simulink model "ACS_PIL"  (R2018b)
settings: Solver=FixedStepDiscrete  StartTime=0.0  StopTime=10000  FixedStep=0.01  MaxStep=10  RelTol=1e-5  AbsTol=1e-5  EnableMultiTasking=on
InitFcn:
  | initialization
values from neighbouring files (symbols this model uses):
  A = [0.25  0.25  0.25  0.25  0.25  0.25]    [initialization.m]
  AE = asin(Re/(Re+h))    [initialization.m]
  air_density = [1.2250e+000  3.8990e-002  1.7740e-002  8.2790e-003  3.9720e-003  1.9950e-003  1.0570e-003                5.8210e-004  3.2060e-004  1.7180e-004  8.7700e-005  4.1780e-005  1.9050e-005  8.3370e-006                3.3960e-006  1.3430e-006  5.2970e-007  9.6610e-008  2.4380e-008  8.4840e-009  3.8450e-009                2.0700e-009  1.2440e-009  5.4640e-010  2.7890e-010  7.2480e-011  2.4180e-011  9.1580 ...(+138 chars)    [initialization.m]
  altitude = [    0       25000       30000       35000       40000       45000       50000       55000             60000       65000       70000       75000       80000       85000       90000       95000            100000      110000      120000      130000      140000      150000      160000      180000            200000      250000      300000      350000      400000      450000      500000      600000     ...(+51 chars)    [initialization.m]
  c_diffus = [0.02   0.02   0.02    0.02    0.02    0.02]    [initialization.m]
  c_spec = [0.02   0.02   0.02    0.02    0.02    0.02]    [initialization.m]
  CD = 2    [initialization.m]
  Cell_Area = 30.18*1e-4    (= 0.003018)    [initialization.m]
  CM_mm01 = [-27723, 1088, -239;  -764, -25026, -219; 1299, -416, -23472]    [attitude_control.m]
  CM_mm02 = [-27799, 42,     95; -1261, -26308,  -43; 2693,  458, -24088]    [attitude_control.m]
  CM_mm03 = [9988,0,0; 0, 9989,0; 0,0,10036]    [attitude_control.m]
  CO_mm01 = [2.5332,  2.5200, 2.4915]    [attitude_control.m]
  CO_mm02 = [2.5348,  2.5260, 2.4664]    [attitude_control.m]
  CO_mm03 = [0.0008, -0.0006, 0.0007]    [attitude_control.m]
  cos50 = cos (50/360*2*pi)    [initialization.m]
  cosines = [0.087 0.174  0.500 0.634 0.866]    [initialization.m]
  dip_coel = acos(g01/H0)    [initialization.m]
  dip_long = atan2(h11,g11)    [initialization.m]
  E_EOL = E_BOL*TD_T*TD_R    (= 0.213003)    [initialization.m]
  H0 = norm([g01,g11,h11])    [initialization.m]
  inc = 1.7231    [initialization.m]
  Inertia_tensor = [2.8  0  0;                   0  2.8  0;                   0  0  2]    [initialization.m]
  K_l = 0.1    [initialization.m]
  kelly = [0.000 0.100  0.450 0.635 0.866]    [initialization.m]
  light_speed = 3e8    (= 300000000)    [initialization.m]
  M_SR = 1377*0.967    (= 1331.559)    [initialization.m]
  MM_Working = [1 1 0]    [attitude_control.m]
  N_B = [  1     0    0,         -1     0    0,          0     1    0,          0    -1    0,          0     0    1,          0     0   -1]    [initialization.m]
  Ncell_Xn = 40    [initialization.m]
  Ncell_Xp = 40    [initialization.m]
  Ncell_Yn = 40    [initialization.m]
  Ncell_Yp = 40    [initialization.m]
  Ncell_Zn = 00    (= 0)    [initialization.m]
  Ncell_Zp = 20    [initialization.m]
  NX = [1 0 0]    [initialization.m]
  NY = [0 1 0]    [initialization.m]
  NZ = [0 0 1]    [initialization.m]
  omega_BI_B0 = [0.1;-0.1;-0.1]    [initialization.m]
  omega_e = 7.29e-5    (= 7.29e-05)    [initialization.m]
  omega_o = (1/r)*(G*M/r)^0.5    (= 0.00108253225434)    [initialization.m]
  quat_0 = E321_to_quat([phi0, theta0, psi0])    [initialization.m]
  r = h + Re    (= 6978137)    [initialization.m]
  r_cm_B = [(0.156e-2 * 42.3 + 0.16917 * 22)/64.3,           (0.248e-1 * 42.3 + -0.35948e-1 * 22)/64.3,           (0.164e-2 * 42.3 + 0.14518e-3 * 22)/64.3]    [initialization.m]
  r_cp_a_B = [0 0 0]    [initialization.m]
  r_cp_s_B = [0 0 0]    [initialization.m]
  RAAN_rt = 2.02e-7    (= 2.02e-07)    [initialization.m]
  Re = 6378137    [initialization.m]
  t0 = 2456738.000000    (= 2456738)    [initialization.m]
  TA_0 = 0    [initialization.m]
  theta_g0 = 0    [initialization.m]
undefined symbols (not defined in the file or in its folder): DiscIntNeverNeededParam, magnitude, serial
libraries: simulink x15, vrlib x3, instrumentlib x3, realtime_pacer_lib x1
(part 1 of 3)
settings Model: Creator=assal  LastModifiedBy=jzamora
settings SolverCC: AutoScaleAbsTol=off  ShapePreserveControl=EnableAll  AutoInsertRateTranBlk=on
settings DataIOCC: SaveFormat=Array  SignalLoggingSaveFormat=ModelDataLogs
settings OptimizationCC: BlockReduction=off  DefaultParameterBehavior=Inlined  BufferReuse=off  ExpressionDepthLimit=2147483647  InitFltsAndDblsToZero=on  LifeSpan=inf
settings DebuggingCC: ArtificialAlgebraicLoopMsg=none  CheckSSInitialOutputMsg=off  UnderspecifiedInitializationDetection=Classic  MergeDetectMultiDrivingBlocksExec=none  BlockPriorityViolationMsg=error  SolverPrmCheckMsg=error  Int32ToFloatConvMsg=none  ParameterPrecisionLossMsg=none  ParameterTunabilityLossMsg=none  FcnCallInpInsideContextMsg=warning  StateNameClashWarn=warning  SFUnexpectedBacktrackingDiag=warning  SFNoUnconditionalDefaultTransitionDiag=warning  SFExecutionAtInitializationDiag=none
settings HardwareCC: ProdBitPerPointer=32  ProdBitPerSizeT=32  ProdBitPerPtrDiffT=32  ProdLargestAtomicFloat=None  ProdIntDivRoundTo=Undefined  ProdEndianess=Unspecified  ProdWordSize=32  ProdHWDeviceType=32-bit Generic
settings ModelReferenceCC: PropagateSignalLabelsOutOfModel=off
settings SFSimCC: SimUseLocalCustomCode=off
settings RTWCC: RTWUseLocalCustomCode=off
settings CodeAppCC: StateflowObjectComments=on
settings GRTTargetCC: TargetLangStandard=C89/C90 (ANSI)  GeneratePreprocessorConditionals=Disable all  CombineOutputUpdateFcns=off  GRTInterface=on
settings ConfigComp: CovMetricSettings=dw  CovHtmlReporting=on  CovSaveCumulativeToWorkspaceVar=on  CovSaveSingleToWorkspaceVar=on  CovExternalEMLEnable=off

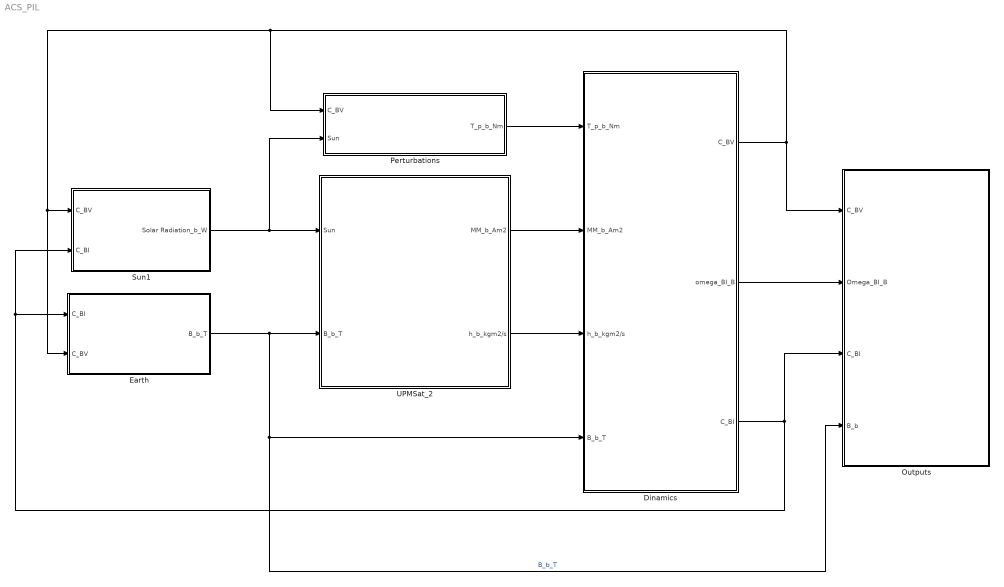
== system ACS_PIL ==
  Dinamics : Subsystem
  Earth : Subsystem
  Outputs : Subsystem
  Perturbations : Subsystem
  Sun1 : Subsystem
  UPMSat_2 : Subsystem
  wires:
  Earth/1(B_b_T) -> Outputs/4(B_b), Dinamics/4(B_b_T), UPMSat_2/2(B_b_T)  "B_b_T"
  Sun1/1(Solar Radiation_b_W) -> Perturbations/2(Sun), UPMSat_2/1(Sun)
  UPMSat_2/1(MM_b_Am2) -> Dinamics/2(MM_b_Am2)
  Perturbations/1(T_p_b_Nm) -> Dinamics/1(T_p_b_Nm)
  Dinamics/1(C_BV) -> Earth/2(C_BV), Sun1/1(C_BV), Perturbations/1(C_BV), Outputs/1(C_BV)
  Dinamics/2(omega_BI_B) -> Outputs/2(Omega_BI_B)
  Dinamics/3(C_BI) -> Outputs/3(C_BI), Earth/1(C_BI), Sun1/2(C_BI)
  UPMSat_2/2(h_b_kgm2/s) -> Dinamics/3(h_b_kgm2/s)

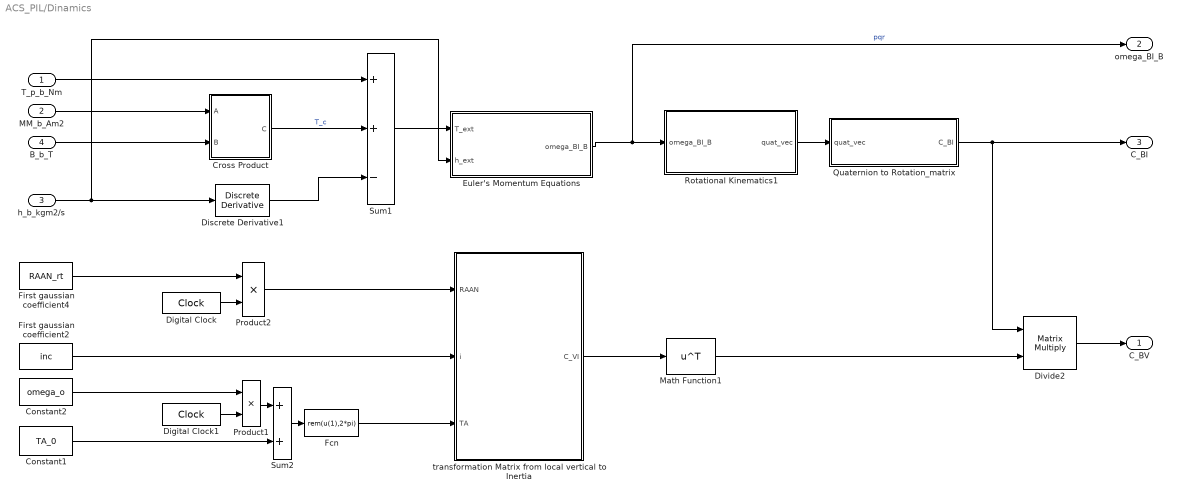
== system ACS_PIL/Dinamics ==
  T_p_b_Nm : Inport
  MM_b_Am2 : Inport  Port=2
  h_b_kgm2/s : Inport  Port=3
  B_b_T : Inport  Port=4
  " First gaussian coefficient2" : Constant  Value=inc
  " First gaussian coefficient4" : Constant  Value=RAAN_rt
  Constant1 : Constant  Value=TA_0
  Constant2 : Constant  Value=omega_o
  Cross Product : Subsystem
  Digital Clock : DigitalClock  SampleTime=0.01
  Digital Clock1 : DigitalClock  SampleTime=0.01
  Discrete Derivative1 : simulink/Discrete/Discrete Derivative  gainval=1.0  ICPrevScaledInput=0.0  OutMin=[]  OutMax=[]  OutDataType=fixdt(1, 16)  OutScaling=2^-10  DoSatur=off
  Divide2 : Product  Inputs=**  Multiplication=Matrix(*)
  Euler's Momentum Equations : Subsystem
  Fcn : Fcn  Expr=rem(u(1),2*pi)
  Math Function1 : Math  Operator=transpose  SaturateOnIntegerOverflow=on
  Product1 : Product  RndMeth=Zero
  Product2 : Product  RndMeth=Zero
  Quaternion to Rotation_matrix : Subsystem
  Rotational Kinematics1 : Subsystem
  Sum1 : Sum  Inputs=++-
  Sum2 : Sum
  transformation Matrix from local vertical to Inertia : Subsystem
  C_BV : Outport
  omega_BI_B : Outport  Port=2
  C_BI : Outport  Port=3
  wires:
  T_p_b_Nm/1 -> Sum1/1
  Sum1/1 -> Euler's Momentum Equations/1(T_ext)
  Euler's Momentum Equations/1(omega_BI_B) -> Rotational Kinematics1/1(omega_BI_B), omega_BI_B/1  "pqr"
  B_b_T/1 -> Cross Product/2(B)
  MM_b_Am2/1 -> Cross Product/1(A)
  Cross Product/1(C) -> Sum1/2  "T_c"
  h_b_kgm2/s/1 -> Discrete Derivative1/1, Euler's Momentum Equations/2(h_ext)
  Rotational Kinematics1/1(quat_vec) -> Quaternion to Rotation_matrix/1(quat_vec)
  Quaternion to Rotation_matrix/1(C_BI) -> Divide2/1, C_BI/1
  Constant2/1 -> Product1/1
  Digital Clock1/1 -> Product1/2
  Product1/1 -> Sum2/1
  Constant1/1 -> Sum2/2
  Sum2/1 -> Fcn/1
  Fcn/1 -> transformation Matrix from local vertical to Inertia/3(TA)
  " First gaussian coefficient4"/1 -> Product2/1
  Digital Clock/1 -> Product2/2
  Product2/1 -> transformation Matrix from local vertical to Inertia/1(RAAN)
  " First gaussian coefficient2"/1 -> transformation Matrix from local vertical to Inertia/2(i)
  transformation Matrix from local vertical to Inertia/1(C_VI) -> Math Function1/1
  Divide2/1 -> C_BV/1
  Math Function1/1 -> Divide2/2
  Discrete Derivative1/1 -> Sum1/3

== system ACS_PIL/Earth ==
  C_BI : Inport
  C_BV : Inport  Port=2
  " First gaussian coefficient1" : Constant  Value=dip_coel
  " First gaussian coefficient3" : Constant  Value=dip_long
  " average rotation rate of the Earth" : Constant  Value=omega_e
  Digital Clock1 : DigitalClock  SampleTime=0.01
  Product5 : Product  RndMeth=Zero
  Simple model of Earth's Magnetic Field1 : Subsystem
  Sum2 : Sum
  greenwich sidereal time : Constant  Value=theta_g0
  transformation Matrix fromEarth Centered to Inertia : Subsystem
  B_b_T : Outport
  wires:
  Digital Clock1/1 -> Product5/1
  transformation Matrix fromEarth Centered to Inertia/1(C_ECEFI) -> Simple model of Earth's Magnetic Field1/5(C_ECEFI)
  greenwich sidereal time/1 -> Sum2/1
  Product5/1 -> Sum2/2
  Sum2/1 -> transformation Matrix fromEarth Centered to Inertia/1(dalpha_g)
  " average rotation rate of the Earth"/1 -> Product5/2
  " First gaussian coefficient3"/1 -> Simple model of Earth's Magnetic Field1/4(phi_md)
  " First gaussian coefficient1"/1 -> Simple model of Earth's Magnetic Field1/3(teta_md)
  Simple model of Earth's Magnetic Field1/1(B_b_T) -> B_b_T/1
  C_BI/1 -> Simple model of Earth's Magnetic Field1/1(C_BI)
  C_BV/1 -> Simple model of Earth's Magnetic Field1/2(C_BV)

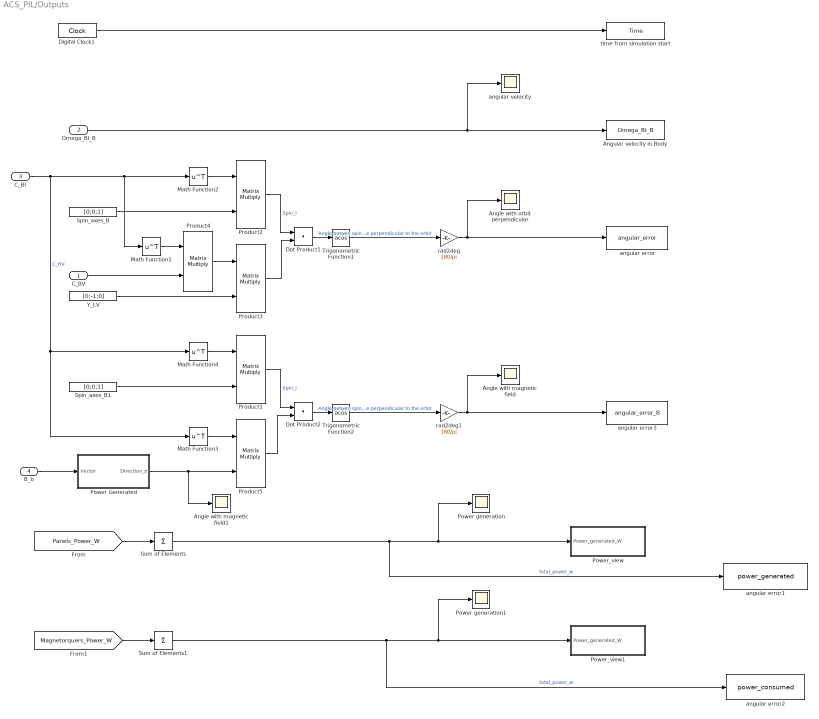
== system ACS_PIL/Outputs ==
  C_BV : Inport
  Omega_BI_B : Inport  Port=2
  C_BI : Inport  Port=3
  B_b : Inport  Port=4
  Angle with magnetic field : Scope
  Angle with magnetic field1 : Scope
  Angle with orbit perpendicular : Scope
  Angular velocity in Body : ToWorkspace  VariableName=Omega_BI_B  SampleTime=-1
      settings: Decimation=1000
  Digital Clock1 : DigitalClock  SampleTime=0.01
  Dot Product1 : DotProduct  InputSameDT=on  OutDataTypeStr=Inherit: Inherit via internal rule
  Dot Product2 : DotProduct  InputSameDT=on  OutDataTypeStr=Inherit: Inherit via internal rule
  Math Function{1..4} (4 alike) : Math  Operator=transpose  SaturateOnIntegerOverflow=on
  Power Generated : Subsystem
  Power generation : Scope
  Power generation1 : Scope
  Power_view : Subsystem
  Power_view1 : Subsystem
  Product{1..5} (5 alike) : Product  Multiplication=Matrix(*)  RndMeth=Zero
  Spin_axes_B : Constant  Value=[0;0;1]
  Spin_axes_B1 : Constant  Value=[0;0;1]
  Sum of Elements : Sum  Inputs=+
  Sum of Elements1 : Sum  Inputs=+
  Trigonometric Function1 : Trigonometry  Operator=acos
  Trigonometric Function2 : Trigonometry  Operator=acos
  Y_LV : Constant  Value=[0;-1;0]
  angular error : ToWorkspace  VariableName=angular_error  SampleTime=-1
      settings: Decimation=1000
  angular error1 : ToWorkspace  VariableName=power_generated  SampleTime=-1
      settings: Decimation=1000
  angular error2 : ToWorkspace  VariableName=power_consumed  SampleTime=-1
      settings: Decimation=1000
  angular error3 : ToWorkspace  VariableName=angular_error_B  SampleTime=-1
      settings: Decimation=1000
  angular velocity : Scope
  rad2deg : Gain  Gain=180/pi
  rad2deg1 : Gain  Gain=180/pi
  time from simulation start : ToWorkspace  VariableName=Time  SampleTime=-1
      settings: Decimation=1000
  wires:
  C_BI/1 -> Math Function3/1, Math Function4/1, Math Function1/1, Math Function2/1  "C_BV"
  Spin_axes_B/1 -> Product2/2
  Product2/1 -> Dot Product1/1  "Spin_I"
  Dot Product1/1 -> Trigonometric Function1/1
  Trigonometric Function1/1 -> rad2deg/1  "Angle betwen spin and the perpendicular to the orbit"
  rad2deg/1 -> angular error/1, Angle with orbit perpendicular/1
  [Panels_Power_W] -> Sum of Elements/1
  Sum of Elements/1 -> angular error1/1, Power generation/1, Power_view/1(Power_generated_W)  "total_power_w"
  Digital Clock1/1 -> time from simulation start/1
  Omega_BI_B/1 -> angular velocity/1, Angular velocity in Body/1
  Math Function2/1 -> Product2/1
  Product3/1 -> Dot Product1/2
  C_BV/1 -> Product4/2
  Math Function1/1 -> Product4/1
  Product4/1 -> Product3/1
  Y_LV/1 -> Product3/2
  [Magnetorquers_Power_W] -> Sum of Elements1/1
  Sum of Elements1/1 -> angular error2/1, Power_view1/1(Power_generated_W), Power generation1/1  "total_power_w"
  Spin_axes_B1/1 -> Product1/2
  Product1/1 -> Dot Product2/1  "Spin_I"
  Dot Product2/1 -> Trigonometric Function2/1
  Trigonometric Function2/1 -> rad2deg1/1  "Angle betwen spin and the perpendicular to the orbit"
  rad2deg1/1 -> Angle with magnetic field/1, angular error3/1
  Math Function4/1 -> Product1/1
  Product5/1 -> Dot Product2/2
  B_b/1 -> Power Generated/1(Vector)
  Math Function3/1 -> Product5/1
  Power Generated/1(Direction_b) -> Angle with magnetic field1/1, Product5/2

== system ACS_PIL/Perturbations ==
  C_BV : Inport
  Sun : Inport  Port=2
  Aerodinamic_Torque : Subsystem
  Gain : Gain
  Gain1 : Gain
  Gain2 : Gain
  Gravity Gradient Torque : Subsystem
  Sum1 : Sum  Inputs=3
  perturbation_Torque1 : Subsystem
  T_p_b_Nm : Outport
  wires:
  Gravity Gradient Torque/1(Tg_B) -> Gain/1
  Aerodinamic_Torque/1(Ta_B) -> Gain1/1
  Gain/1 -> Sum1/1
  Gain1/1 -> Sum1/2
  C_BV/1 -> Aerodinamic_Torque/1(C_BV), Gravity Gradient Torque/1(C_BV)
  Sun/1 -> perturbation_Torque1/1(S_ES_B)
  Sum1/1 -> T_p_b_Nm/1  "T_perturbation_b_Nm"
  perturbation_Torque1/1(Ts_B) -> Gain2/1
  Gain2/1 -> Sum1/3

== system ACS_PIL/Sun1 ==
  C_BV : Inport
  C_BI : Inport  Port=2
  Bus Creator : BusCreator  Inputs=2
  Digital Clock1 : DigitalClock  SampleTime=0.01
  Gain : Gain  Gain=pi/180
  Gain1 : Gain  Gain=pi/180
  Gain2 : Gain  Gain=pi/180
  Min Solar Constant W : Constant  Value=M_SR
  Solar Rays Direction : Subsystem
  Sun Annalema : Subsystem
  Solar Radiation_b_W : Outport
  wires:
  Digital Clock1/1 -> Sun Annalema/1(clock)
  Sun Annalema/2(EOT_deg) -> Gain1/1  "EOT_deg"
  Sun Annalema/3(declination_deg) -> Gain2/1  "declination_deg"
  Gain1/1 -> Solar Rays Direction/3(epsilon)  "EOT_rad"
  Gain2/1 -> Solar Rays Direction/4(delta)  "declination_rad"
  Sun Annalema/1(gamma_deg) -> Gain/1
  Gain/1 -> Solar Rays Direction/2(gamma)
  C_BV/1 -> Solar Rays Direction/5(C_BV)
  Min Solar Constant W/1 -> Solar Rays Direction/1(Solar_const)
  Solar Rays Direction/2(Eclipse) -> Bus Creator/2  "eclipse"
  Solar Rays Direction/1(Sun_b_W) -> Bus Creator/1  "sun_b_W"
  Bus Creator/1 -> Solar Radiation_b_W/1
  C_BI/1 -> Solar Rays Direction/6(C_BI)

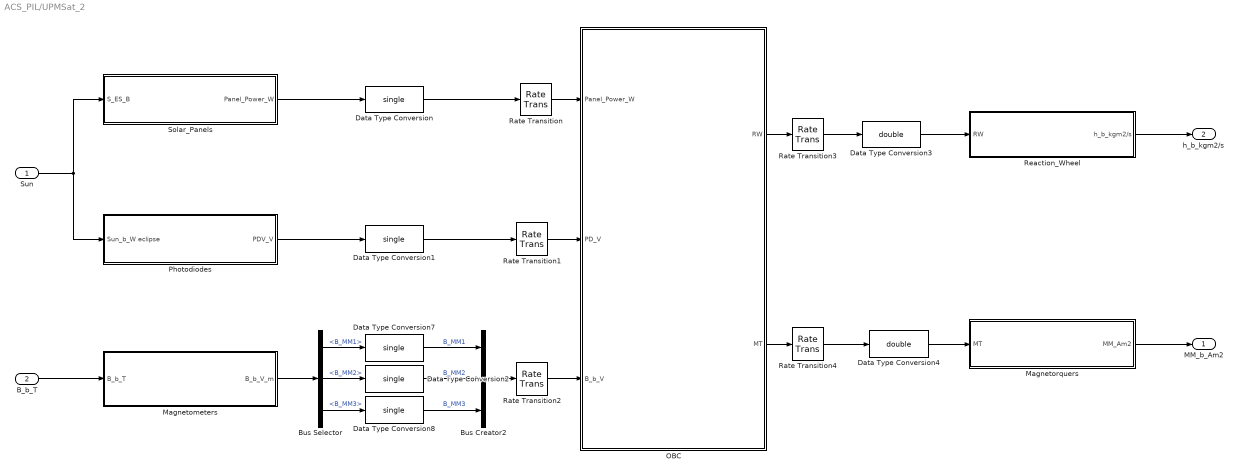
== system ACS_PIL/UPMSat_2 ==
  Sun : Inport
  B_b_T : Inport  Port=2
  Bus Creator2 : BusCreator  Inputs=3
  Bus Selector : BusSelector  OutputSignals=B_MM1,B_MM2,B_MM3
  Data Type Conversion{,1..2,7..8} (5 alike) : DataTypeConversion  OutDataTypeStr=single
  Data Type Conversion3 : DataTypeConversion  OutDataTypeStr=double
  Data Type Conversion4 : DataTypeConversion  OutDataTypeStr=double
  Magnetometers : Subsystem
  Magnetorquers : Subsystem
  OBC : Subsystem
  Photodiodes : Subsystem
  Rate Transition : RateTransition  OutPortSampleTime=0.1
  Rate Transition1 : RateTransition  OutPortSampleTime=0.1
  Rate Transition2 : RateTransition  OutPortSampleTime=0.1
  Rate Transition3 : RateTransition  OutPortSampleTime=0.01
  Rate Transition4 : RateTransition  OutPortSampleTime=0.01
  Reaction_Wheel : Subsystem
  Solar_Panels : Subsystem
  MM_b_Am2 : Outport
  h_b_kgm2/s : Outport  Port=2
  wires:
  Sun/1 -> Solar_Panels/1(S_ES_B), Photodiodes/1(Sun_b_W eclipse)
  Solar_Panels/1(Panel_Power_W) -> Data Type Conversion/1
  Photodiodes/1(PDV_V) -> Data Type Conversion1/1
  Magnetometers/1(B_b_V_m) -> Bus Selector/1
  Reaction_Wheel/1(h_b_kgm2/s) -> h_b_kgm2/s/1
  Magnetorquers/1(MM_Am2) -> MM_b_Am2/1
  B_b_T/1 -> Magnetometers/1(B_b_T)
  Data Type Conversion/1 -> Rate Transition/1
  Data Type Conversion1/1 -> Rate Transition1/1
  Bus Selector/1 -> Data Type Conversion7/1  "<B_MM1>"
  Bus Selector/2 -> Data Type Conversion2/1  "<B_MM2>"
  Bus Selector/3 -> Data Type Conversion8/1  "<B_MM3>"
  Data Type Conversion2/1 -> Bus Creator2/2  "B_MM2"
  Data Type Conversion8/1 -> Bus Creator2/3  "B_MM3"
  Data Type Conversion7/1 -> Bus Creator2/1  "B_MM1"
  Bus Creator2/1 -> Rate Transition2/1
  Data Type Conversion3/1 -> Reaction_Wheel/1(RW)
  Data Type Conversion4/1 -> Magnetorquers/1(MT)
  OBC/2(MT) -> Rate Transition4/1
  OBC/1(RW) -> Rate Transition3/1
  Rate Transition/1 -> OBC/1(Panel_Power_W)
  Rate Transition1/1 -> OBC/2(PD_V)
  Rate Transition2/1 -> OBC/3(B_b_V)
  Rate Transition3/1 -> Data Type Conversion3/1
  Rate Transition4/1 -> Data Type Conversion4/1

== system ACS_PIL/Dinamics/Cross Product ==
  A : Inport
  B : Inport  Port=2
  Cross Product : Fcn  Expr=u(2)*u(6)-u(3)*u(5)
  Cross Product1 : Fcn  Expr=u(3)*u(4)-u(1)*u(6)
  Cross Product2 : Fcn  Expr=u(1)*u(5)-u(2)*u(4)
  Mux : Mux  Inputs=2
  Mux1 : Mux  Inputs=3
  C : Outport
  wires:
  A/1 -> Mux/1
  B/1 -> Mux/2
  Mux1/1 -> C/1
  Mux/1 -> Cross Product2/1, Cross Product1/1, Cross Product/1
  Cross Product1/1 -> Mux1/2
  Cross Product2/1 -> Mux1/3
  Cross Product/1 -> Mux1/1

== system ACS_PIL/Dinamics/Euler's Momentum Equations ==
  T_ext : Inport
  h_ext : Inport  Port=2
  Add1 : Sum  Inputs=-+
  Add2 : Sum  Inputs=2
  Constant : Constant  Value=Inertia_tensor  VectorParams1D=off
  Constant1 : Constant  Value=omega_BI_B0  VectorParams1D=off
  Cross Product : Subsystem
  Discrete-Time Integrator : DiscreteIntegrator  InitialConditionSource=external  SampleTime=0.01  ICPrevOutput=DiscIntNeverNeededParam  ICPrevScaledInput=DiscIntNeverNeededParam
  Product : Product  Inputs=/  Multiplication=Matrix(*)
  Product1 : Product  Multiplication=Matrix(*)  RndMeth=Zero
  Product2 : Product  Multiplication=Matrix(*)  RndMeth=Zero
  omega_BI_B : Outport
  wires:
  Product1/1 -> Add2/1  "I * omega_BI_B"
  Product2/1 -> Discrete-Time Integrator/1  "omega_BI_B_dot"
  Add1/1 -> Product2/2
  Product/1 -> Product2/1
  T_ext/1 -> Add1/2
  Cross Product/1(C) -> Add1/1
  Discrete-Time Integrator/1 -> Cross Product/1(A), Product1/2, omega_BI_B/1  "omega_BI_B"
  Constant/1 -> Product/1, Product1/1
  Add2/1 -> Cross Product/2(B)
  h_ext/1 -> Add2/2
  Constant1/1 -> Discrete-Time Integrator/2

== system ACS_PIL/Dinamics/Quaternion to Rotation_matrix ==
  quat_vec : Inport
  Fcn : Fcn  Expr=1-2*(u(2)^2+u(3)^2)
  Fcn1 : Fcn  Expr=2*(u(1)*u(2)-u(3)*u(4))
  Fcn2 : Fcn  Expr=2*(u(1)*u(3)+u(2)*u(4))
  Fcn3 : Fcn  Expr=2*(u(1)*u(2)+u(3)*u(4))
  Fcn4 : Fcn  Expr=1-2*(u(1)^2+u(3)^2)
  Fcn5 : Fcn  Expr=2*(u(2)*u(3)-u(4)*u(1))
  Fcn6 : Fcn  Expr=2*(u(1)*u(3)-u(4)*u(2))
  Fcn7 : Fcn  Expr=2*(u(2)*u(3)+u(4)*u(1))
  Fcn8 : Fcn  Expr=1-2*(u(1)^2+u(2)^2)
  Mux : Mux  Inputs=9
  Reshape : Reshape  OutputDimensionality=Customize  OutputDimensions=[3,3]
  C_BI : Outport
  wires:
  Reshape/1 -> C_BI/1
  Mux/1 -> Reshape/1
  Fcn8/1 -> Mux/9
  Fcn7/1 -> Mux/8
  Fcn6/1 -> Mux/7
  Fcn5/1 -> Mux/6
  Fcn4/1 -> Mux/5
  Fcn3/1 -> Mux/4
  Fcn2/1 -> Mux/3
  Fcn1/1 -> Mux/2
  Fcn/1 -> Mux/1
  quat_vec/1 -> Fcn8/1, Fcn7/1, Fcn6/1, Fcn5/1, Fcn4/1, Fcn3/1, Fcn2/1, Fcn1/1, Fcn/1

== system ACS_PIL/Dinamics/Rotational Kinematics1 ==
  omega_BI_B : Inport
  4*4 Skew Mtrix of a 3*1 vector : Subsystem
  Constant : Constant  Value=quat_0
  Constant1 : Constant
  Constant2 : Constant  Value=K_l
  Discrete-Time Integrator : DiscreteIntegrator  InitialConditionSource=external  SampleTime=0.01  ICPrevOutput=DiscIntNeverNeededParam  ICPrevScaledInput=DiscIntNeverNeededParam
  Divide1 : Product  Inputs=*/
  Divide3 : Product  Inputs=3
  Gain : Gain  Gain=1/2
  Math Function : Math  Operator=magnitude^2  SaturateOnIntegerOverflow=on
  Product : Product  Multiplication=Matrix(*)  RndMeth=Zero
  Quaternion Norm : Subsystem  AncestorBlock=aerolibutil/Quaternion Norm  mask(Quaternion Norm){}
      mask help: Calculate the norm of a quaternion.
      mask Help: web(asbhelp);
  Quaternion Norm1 : Subsystem  AncestorBlock=aerolibutil/Quaternion Norm  mask(Quaternion Norm){}
      mask help: Calculate the norm of a quaternion.
      mask Help: web(asbhelp);
  Sum : Sum  Inputs=+-
  Sum2 : Sum
  quat_vec : Outport
  wires:
  Quaternion Norm1/1(norm(q)) -> Math Function/1
  Divide1/1 -> Quaternion Norm1/1(q), Divide3/2, Product/2, quat_vec/1
  Divide3/1 -> Sum2/2
  Gain/1 -> Sum2/1
  Constant2/1 -> Divide3/1
  Sum2/1 -> Discrete-Time Integrator/1
  Constant/1 -> Discrete-Time Integrator/2
  Sum/1 -> Divide3/3  "epsilon_t"
  Math Function/1 -> Sum/2
  Constant1/1 -> Sum/1
  Product/1 -> Gain/1
  Quaternion Norm/1(norm(q)) -> Divide1/2
  omega_BI_B/1 -> 4*4 Skew Mtrix of a 3*1 vector/1(omega)
  Discrete-Time Integrator/1 -> Divide1/1, Quaternion Norm/1(q)
  4*4 Skew Mtrix of a 3*1 vector/1(4*4 omega_skew matrix1) -> Product/1

== system ACS_PIL/Dinamics/transformation Matrix from local vertical to Inertia ==
  RAAN : Inport
  i : Inport  Port=2
  TA : Inport  Port=3
  Inertial 2 Orbital Plane1 : Subsystem
  Orbital Reference 2 Local Vertical1 : Subsystem
  Product : Product  Multiplication=Matrix(*)  RndMeth=Zero
  Product1 : Product  Multiplication=Matrix(*)  RndMeth=Zero
  C_VI : Outport
  wires:
  Inertial 2 Orbital Plane1/1(C_OPROPF) -> Product/2  "C_OPROPF"
  Orbital Reference 2 Local Vertical1/1(C_VOPR) -> Product/1  "C_VOPR"
  TA/1 -> Inertial 2 Orbital Plane1/3(TA)
  RAAN/1 -> Inertial 2 Orbital Plane1/2(RAAN)
  i/1 -> Inertial 2 Orbital Plane1/1(i)
  Product/1 -> Product1/1
  Product1/1 -> C_VI/1
  Inertial 2 Orbital Plane1/2(C_OPFI) -> Product1/2  "C_OPFI"

== system ACS_PIL/Earth/Simple model of Earth's Magnetic Field1 ==
  C_BI : Inport
  C_BV : Inport  Port=2
  teta_md : Inport  Port=3
  phi_md : Inport  Port=4
  C_ECEFI : Inport  Port=5
  Demux : Demux  Outputs=2
  Divide1 : Product  Inputs=**  Multiplication=Matrix(*)
  Divide10 : Product  Inputs=**  Multiplication=Matrix(*)
  Math Function1 : Math  Operator=transpose  SaturateOnIntegerOverflow=on
  Math Function2 : Math  Operator=transpose  SaturateOnIntegerOverflow=on
  Product1 : Product  Multiplication=Matrix(*)  RndMeth=Zero
  Product4 : Product  Inputs=3  Multiplication=Matrix(*)  RndMeth=Zero
  Simple model of Earth's Magnetic Field1 : Subsystem
  earth_sat vector in local vertical reference system : Constant  Value=[0 ;0 ;-r]  VectorParams1D=off
  longitude_latitude : Subsystem
  B_b_T : Outport
  wires:
  teta_md/1 -> Simple model of Earth's Magnetic Field1/3(teta_md)
  phi_md/1 -> Simple model of Earth's Magnetic Field1/4(phi_md)
  longitude_latitude/1(long_lat) -> Demux/1
  Demux/1 -> Simple model of Earth's Magnetic Field1/1(long)
  Demux/2 -> Simple model of Earth's Magnetic Field1/2(lat)
  earth_sat vector in local vertical reference system/1 -> Divide10/2  "R_LV"
  Divide10/1 -> longitude_latitude/1(R_ECEF)  "R_ECEF"
  Product4/1 -> Divide10/1  "C_ECEFV"
  C_BV/1 -> Product4/3
  Math Function2/1 -> Product4/2
  C_BI/1 -> Math Function2/1, Product1/1
  Divide1/1 -> B_b_T/1
  C_ECEFI/1 -> Math Function1/1, Product4/1
  Product1/1 -> Divide1/1  "C_BECEF"
  Simple model of Earth's Magnetic Field1/1(B_ECEF_T) -> Divide1/2
  Math Function1/1 -> Product1/2

== system ACS_PIL/Earth/transformation Matrix fromEarth Centered to Inertia ==
  dalpha_g : Inport
  Constant{1,4..5,8} (4 alike) : Constant  Value=0
  Constant6 : Constant
  Gain : Gain  Gain=-1
  Mux : Mux  Inputs=9
  Reshape : Reshape  OutputDimensionality=Customize  OutputDimensions=[3,3]
  Trigonometric Function : Trigonometry  Operator=cos
  Trigonometric Function1 : Trigonometry
  C_ECEFI : Outport
  wires:
  Mux/1 -> Reshape/1
  Trigonometric Function1/1 -> Gain/1, Mux/4
  Constant1/1 -> Mux/3
  Constant5/1 -> Mux/6
  Constant8/1 -> Mux/7
  Constant4/1 -> Mux/8
  Constant6/1 -> Mux/9
  Reshape/1 -> C_ECEFI/1
  Trigonometric Function/1 -> Mux/1, Mux/5
  dalpha_g/1 -> Trigonometric Function1/1, Trigonometric Function/1
  Gain/1 -> Mux/2

== system ACS_PIL/Outputs/Power Generated ==
  Vector : Inport
  Add : Sum  Inputs=+++
  Add1 : Sum  Inputs=2
  Compare To Zero : simulink/Logic and Bit Operations/Compare To Zero  relop===  OutDataTypeStr=uint8  ZeroCross=off
  Demux : Demux  Outputs=3
  Math Function : Math  Operator=magnitude^2  SaturateOnIntegerOverflow=on
  Math Function1 : Math  Operator=magnitude^2  SaturateOnIntegerOverflow=on
  Math Function2 : Math  Operator=magnitude^2  SaturateOnIntegerOverflow=on
  Math Function3 : Math  Operator=sqrt  SaturateOnIntegerOverflow=on
  Product4 : Product  Inputs=*/  RndMeth=Zero
  Direction_b : Outport
  wires:
  Demux/1 -> Math Function/1
  Demux/2 -> Math Function1/1
  Math Function/1 -> Add/1
  Math Function1/1 -> Add/2
  Add/1 -> Math Function3/1
  Math Function3/1 -> Add1/1, Compare To Zero/1
  Demux/3 -> Math Function2/1
  Math Function2/1 -> Add/3
  Vector/1 -> Product4/1, Demux/1
  Product4/1 -> Direction_b/1
  Add1/1 -> Product4/2
  Compare To Zero/1 -> Add1/2

== system ACS_PIL/Outputs/Power_view ==
  Power_generated_W : Inport
  Discrete-Time Integrator : DiscreteIntegrator  SampleTime=0.01  ICPrevOutput=DiscIntNeverNeededParam  ICPrevScaledInput=DiscIntNeverNeededParam
  Product : Product  Inputs=*/  RndMeth=Zero
  Ramp : simulink/Sources/Ramp  slope=1  start=0  InitialOutput=0.001
  Terminator1 : Terminator
  wires:
  Discrete-Time Integrator/1 -> Product/1
  Ramp/1 -> Product/2
  Power_generated_W/1 -> Discrete-Time Integrator/1
  Product/1 -> Terminator1/1

== system ACS_PIL/Outputs/Power_view1 ==
  Power_generated_W : Inport
  Discrete-Time Integrator : DiscreteIntegrator  SampleTime=0.01  ICPrevOutput=DiscIntNeverNeededParam  ICPrevScaledInput=DiscIntNeverNeededParam
  Product : Product  Inputs=*/  RndMeth=Zero
  Ramp : simulink/Sources/Ramp  slope=1  start=0  InitialOutput=0.001
  Terminator1 : Terminator
  wires:
  Product/1 -> Terminator1/1
  Power_generated_W/1 -> Discrete-Time Integrator/1
  Ramp/1 -> Product/2
  Discrete-Time Integrator/1 -> Product/1

== system ACS_PIL/Perturbations/Aerodinamic_Torque ==
  C_BV : Inport
  Add3 : Sum  Inputs=+-
  Aerodynamic : Subsystem
  Earth's radius : Constant  Value=Re
  Subsystem : Subsystem
  air_density1 : Lookup  InputValues=altitude  Table=air_density
  r_sat : Constant  Value=r
  Ta_B : Outport
  wires:
  Subsystem/1(v_vec_b) -> Aerodynamic/1(v_B)
  r_sat/1 -> Add3/1
  Earth's radius/1 -> Add3/2
  Add3/1 -> air_density1/1
  air_density1/1 -> Aerodynamic/2(air_density)
  C_BV/1 -> Subsystem/1(C_BV)
  Aerodynamic/1(Ta_B) -> Ta_B/1

== system ACS_PIL/Perturbations/Gravity Gradient Torque ==
  C_BV : Inport
  Constant1 : Constant  Value=Inertia_tensor
  Constant2 : Constant  Value=omega_o
  Constant4 : Constant  Value=3  VectorParams1D=off
  Cross Product : vrlib/Utilities/Cross Product
      settings: SourceProductBaseCode=VR
  Divide : Product  Inputs=***
  Math Function : Math  Operator=square  SaturateOnIntegerOverflow=on
  Product : Product  Multiplication=Matrix(*)  RndMeth=Zero
  Product1 : Product  Multiplication=Matrix(*)  RndMeth=Zero
  sat_earth vector in local vertical reference system : Constant  Value=[0 ;0 ;1]  VectorParams1D=off
  Tg_B : Outport
  wires:
  Math Function/1 -> Divide/3
  Constant2/1 -> Math Function/1
  Divide/1 -> Tg_B/1
  Cross Product/1 -> Divide/1
  Product/1 -> Cross Product/2
  sat_earth vector in local vertical reference system/1 -> Product1/2
  C_BV/1 -> Product1/1
  Product1/1 -> Cross Product/1, Product/2
  Constant1/1 -> Product/1
  Constant4/1 -> Divide/2

== system ACS_PIL/Perturbations/perturbation_Torque1 ==
  S_ES_B : Inport
  Bus Selector : BusSelector  OutputSignals=sun_b_W,eclipse
  Power Generated : Subsystem
  Solar Torque and Force Calculation : Subsystem
  Ts_B : Outport
  wires:
  Bus Selector/2 -> Solar Torque and Force Calculation/3(eclipse)  "<eclipse>"
  Power Generated/2(Solar_Flux_W) -> Solar Torque and Force Calculation/2(Solar_const)
  Power Generated/1(Solar_Direction_b) -> Solar Torque and Force Calculation/1(S_ES_B)
  S_ES_B/1 -> Bus Selector/1
  Bus Selector/1 -> Power Generated/1(Sol_b_W)  "<sun_b_W>"
  Solar Torque and Force Calculation/1(Ts_B) -> Ts_B/1

== system ACS_PIL/Sun1/Solar Rays Direction ==
  Solar_const : Inport
  gamma : Inport  Port=2
  epsilon : Inport  Port=3
  delta : Inport  Port=4
  C_BV : Inport  Port=5
  C_BI : Inport  Port=6
  Divide1 : Product  Inputs=**  Multiplication=Matrix(*)
  Eclipse_ : Subsystem
  Logical Operator : Logic  Operator=NOT  AllPortsSameDT=off  OutDataTypeStr=boolean
  Product8 : Product  RndMeth=Zero
  Solar direction in inertial : Subsystem
  Sun_b_W : Outport
  Eclipse : Outport  Port=2
  wires:
  C_BV/1 -> Eclipse_/2(C_BV)
  Solar direction in inertial/1(S_ES_I) -> Divide1/2
  gamma/1 -> Solar direction in inertial/3(gamma)
  epsilon/1 -> Solar direction in inertial/2(epsilon)
  delta/1 -> Solar direction in inertial/1(delta)
  Solar_const/1 -> Product8/1
  Eclipse_/1(eclipse) -> Logical Operator/1
  Logical Operator/1 -> Eclipse/1
  Divide1/1 -> Eclipse_/1(Earth-Sun B), Product8/2  "Solar radiation direction in body"
  Product8/1 -> Sun_b_W/1
  C_BI/1 -> Divide1/1

== system ACS_PIL/Sun1/Sun Annalema ==
  clock : Inport
  Calculating Sun position : Subsystem  mask(Calculating sun position){}
      mask help:
      | This block calculates the coordinates of the Sun following the specifications in "The astronomical Almanac for the year 2008" in section C24
      | This formulas have a precision of 0.1 minutes from 1950 to 2050.
      |
      | Mean longitude (gamma angle) which is the angle between Vernal equinox and Mean Sun
      | vector. This angle is zero at vernal equiniox (22th of March) and reaches 360deg after a year.
      |
      | Declination (delta) is the angle of the sun respect to the ecuatorial plane of the Earth.
      |
      | Equation of time is the apparent time of the sun minus the mean time (*4 in degrees).
  J2000.0 : Constant  Value=2451545.0
  Sum1 : Sum  Inputs=+-
  Sum2 : Sum
  sec to day : Gain  Gain=1/(24*3600)
  t0 : Constant  Value=t0
  gamma_deg : Outport
  EOT_deg : Outport  Port=2
  declination_deg : Outport  Port=3
  wires:
  J2000.0/1 -> Sum1/2
  clock/1 -> sec to day/1
  sec to day/1 -> Sum2/1
  Sum2/1 -> Sum1/1
  t0/1 -> Sum2/2
  Sum1/1 -> Calculating Sun position/1(Time_passed from J2000.0)  "n of days from J2000.0"
  Calculating Sun position/1(gamma_deg) -> gamma_deg/1
  Calculating Sun position/2(EOT_deg) -> EOT_deg/1
  Calculating Sun position/3(declination_deg) -> declination_deg/1

== system ACS_PIL/UPMSat_2/Magnetometers ==
  B_b_T : Inport
  Bus Creator : BusCreator  Inputs=3
  Gain1 : Gain  Gain=1e9
  Magnetometer_1 : Subsystem
  Magnetometer_2 : Subsystem
  Magnetometer_3 : Subsystem
  B_b_V_m : Outport
  wires:
  B_b_T/1 -> Gain1/1
  Magnetometer_1/1(B_b_V_m1) -> Bus Creator/1  "B_MM1"
  Magnetometer_2/1(B_b_V_m1) -> Bus Creator/2  "B_MM2"
  Magnetometer_3/1(B_b_V_m1) -> Bus Creator/3  "B_MM3"
  Bus Creator/1 -> B_b_V_m/1
  Gain1/1 -> Magnetometer_1/1(B_b_nT), Magnetometer_3/1(B_b_nT), Magnetometer_2/1(B_b_nT)  "B_b_nT"

== system ACS_PIL/UPMSat_2/Magnetorquers ==
  MT : Inport
  Demux2 : Demux  Outputs=3
  Gain1 : Gain  Gain=22
  Gain2 : Gain  Gain=22
  Gain3 : Gain  Gain=22
  Magnetorquers1 : Subsystem
  Magnetorquers2 : Subsystem
  Magnetorquers4 : Subsystem
  Mux : Mux  Inputs=3
  Mux1 : Mux  Inputs=3
  Scope : Scope
  MM_Am2 : Outport
  tag scope: Magnetorquers_Power_W=global
  wires:
  Demux2/1 -> Gain3/1
  Demux2/2 -> Gain1/1
  Demux2/3 -> Gain2/1
  Magnetorquers4/1(MM_Am2) -> Scope/1, Mux/1
  Magnetorquers1/1(MM_Am2) -> Mux/2
  Magnetorquers2/1(MM_Am2) -> Mux/3
  Mux/1 -> MM_Am2/1
  MT/1 -> Demux2/1  "total_power_w"
  Magnetorquers4/2(MM_W) -> Mux1/1
  Magnetorquers1/2(MM_W) -> Mux1/2
  Magnetorquers2/2(MM_W) -> Mux1/3
  Mux1/1 -> [Magnetorquers_Power_W]
  Gain3/1 -> Magnetorquers4/1(MT)
  Gain1/1 -> Magnetorquers1/1(MT)
  Gain2/1 -> Magnetorquers2/1(MT)

== system ACS_PIL/UPMSat_2/OBC ==
  Panel_Power_W : Inport
  PD_V : Inport  Port=2
  B_b_V : Inport  Port=3
  Bus Creator : BusCreator  Inputs=2
  Bus Creator1 : BusCreator  Inputs=2
  Bus Selector : BusSelector  OutputSignals=signal1,signal2
  Bus Selector1 : BusSelector  OutputSignals=signal1,signal2,signal3
  Constant3 : Constant  Value=0  OutDataTypeStr=single
  Data Adquisition : Subsystem
  Experimentall Attitude Control : Subsystem
  Nominal Attitude Control : Subsystem
  Terminator1 : Terminator
  RW : Outport
  MT : Outport  Port=2
  wires:
  B_b_V/1 -> Data Adquisition/3(B_b_V)
  Panel_Power_W/1 -> Data Adquisition/1(PP_W)
  PD_V/1 -> Data Adquisition/2(PD_V)
  Data Adquisition/1(PP_UPC) -> Experimentall Attitude Control/1(PP_UPC)
  Data Adquisition/2(PD_UPC) -> Experimentall Attitude Control/2(PD_UPC)
  Nominal Attitude Control/1(MT) -> Bus Creator/1
  Bus Creator1/1 -> Terminator1/1
  Experimentall Attitude Control/1(MT) -> Bus Creator1/1
  Experimentall Attitude Control/2(RW) -> Bus Creator1/2
  Bus Creator/1 -> Bus Selector/1
  Bus Selector/1 -> MT/1  "<signal1>"
  Bus Selector/2 -> RW/1  "<signal2>"
  Constant3/1 -> Bus Creator/2
  Bus Selector1/2 -> Nominal Attitude Control/2(B_b_mm02_UPC)  "<signal2>"
  Bus Selector1/1 -> Nominal Attitude Control/1(B_b_mm01_UPC)  "<signal1>"
  Bus Selector1/3 -> Nominal Attitude Control/3(B_b_mm03_UPC)  "<signal3>"
  Data Adquisition/3(B_b_UPC) -> Experimentall Attitude Control/3(B_b_UPC), Bus Selector1/1

== system ACS_PIL/UPMSat_2/Photodiodes ==
  Sun_b_W eclipse : Inport
  1 Hz2 : DiscretePulseGenerator  PulseType=Time based  PulseWidth=50
  1 Hz3 : DiscretePulseGenerator  PulseType=Time based  Period=0.2  PulseWidth=50  PhaseDelay=1
  Bus Selector : BusSelector  OutputSignals=sun_b_W,eclipse
  Measurements : Subsystem
  Product1 : Product  RndMeth=Zero
  Sun : Subsystem
  Voltage : Subsystem
  PDV_V : Outport
  wires:
  Voltage/1(PD_V) -> Measurements/1(V)
  Sun_b_W eclipse/1 -> Bus Selector/1
  Bus Selector/1 -> Sun/1(Sol_b_W)  "<sun_b_W>"
  Sun/1(Solar_Direction_b) -> Voltage/1(Earth-Sun B)
  Sun/2(Solar_Flux_W) -> Voltage/2(Solar Constant)
  Bus Selector/2 -> Voltage/3(eclipse)  "<eclipse>"
  Product1/1 -> Measurements/Trigger
  Measurements/1(V_V) -> PDV_V/1
  1 Hz3/1 -> Product1/2
  1 Hz2/1 -> Product1/1

== system ACS_PIL/UPMSat_2/Reaction_Wheel ==
  RW : Inport
  Magnetorquer Fil1 : Constant  Value=0  SampleTime=0.01
  Terminator : Terminator
  h_b_kgm2/s : Outport
  wires:
  RW/1 -> Terminator/1
  Magnetorquer Fil1/1 -> h_b_kgm2/s/1

== system ACS_PIL/UPMSat_2/Solar_Panels ==
  S_ES_B : Inport
  3.33 Hz : DiscretePulseGenerator  PulseType=Time based  Period=0.3  PulseWidth=100-1/0.3
  Bus Selector : BusSelector  OutputSignals=sun_b_W,eclipse
  Measurements : Subsystem
  Power : Subsystem
  Power Generated : Subsystem
  Panel_Power_W : Outport
  tag scope: Panels_Power_W=global
  wires:
  Power/1(Power_each_W) -> [Panels_Power_W], Measurements/1(V)
  Bus Selector/1 -> Power Generated/1(Sol_b_W)  "<sun_b_W>"
  Power Generated/1(Solar_Direction_b) -> Power/1(Earth-Sun B)
  Power Generated/2(Solar_Flux_W) -> Power/2(Solar Constant)
  S_ES_B/1 -> Bus Selector/1
  Bus Selector/2 -> Power/3(eclipse)  "<eclipse>"
  3.33 Hz/1 -> Measurements/Trigger
  Measurements/1(V_V) -> Panel_Power_W/1

== system ACS_PIL/Dinamics/Euler's Momentum Equations/Cross Product ==
  A : Inport
  B : Inport  Port=2
  Cross Product : Fcn  Expr=u(2)*u(6)-u(3)*u(5)
  Cross Product1 : Fcn  Expr=u(3)*u(4)-u(1)*u(6)
  Cross Product2 : Fcn  Expr=u(1)*u(5)-u(2)*u(4)
  Mux : Mux  Inputs=2
  Mux1 : Mux  Inputs=3
  C : Outport
  wires:
  A/1 -> Mux/1
  B/1 -> Mux/2
  Mux1/1 -> C/1
  Mux/1 -> Cross Product2/1, Cross Product1/1, Cross Product/1
  Cross Product1/1 -> Mux1/2
  Cross Product2/1 -> Mux1/3
  Cross Product/1 -> Mux1/1

== system ACS_PIL/Dinamics/Rotational Kinematics1/4*4 Skew Mtrix of a 3*1 vector ==
  omega : Inport
  Constant{,1..3} (4 alike) : Constant  Value=0
  Demux : Demux  Outputs=3
  Demux1 : Demux  Outputs=3
  Gain : Gain  Gain=-1
  Mux1 : Mux  Inputs=16
  Reshape : Reshape  OutputDimensionality=Customize  OutputDimensions=[4,4]
  4*4 omega_skew matrix1 : Outport
  wires:
  omega/1 -> Demux/1, Gain/1
  Gain/1 -> Demux1/1
  Constant/1 -> Mux1/1
  Demux1/3 -> Mux1/2, Mux1/12  "-omega_z"
  Demux/2 -> Mux1/3, Mux1/14  "omega_y"
  Demux/3 -> Mux1/15, Mux1/5  "omega_z"
  Constant1/1 -> Mux1/6
  Demux1/1 -> Mux1/4, Mux1/7  "-omega_x"
  Demux1/2 -> Mux1/8, Mux1/9  "-omega_y"
  Demux/1 -> Mux1/10, Mux1/13  "omega_x"
  Constant2/1 -> Mux1/11
  Constant3/1 -> Mux1/16
  Mux1/1 -> Reshape/1
  Reshape/1 -> 4*4 omega_skew matrix1/1

== system ACS_PIL/Dinamics/Rotational Kinematics1/Quaternion Norm ==
  q : Inport
  Demux : Demux
  Math Function : Math  Operator=sqrt  SaturateOnIntegerOverflow=on
  Product{,1..3} (4 alike) : Product
  Sum : Sum  Inputs=4
  norm(q) : Outport
  wires:
  Demux/4 -> Product3/1, Product3/2
  Demux/3 -> Product2/1, Product2/2
  Demux/2 -> Product1/1, Product1/2
  Demux/1 -> Product/1, Product/2
  Product3/1 -> Sum/4
  Product2/1 -> Sum/3
  Product1/1 -> Sum/2
  Product/1 -> Sum/1
  Sum/1 -> Math Function/1
  q/1 -> Demux/1
  Math Function/1 -> norm(q)/1

== system ACS_PIL/Dinamics/Rotational Kinematics1/Quaternion Norm1 ==
  q : Inport
  Demux : Demux
  Math Function : Math  Operator=sqrt  SaturateOnIntegerOverflow=on
  Product{,1..3} (4 alike) : Product
  Sum : Sum  Inputs=4
  norm(q) : Outport
  wires:
  Math Function/1 -> norm(q)/1
  q/1 -> Demux/1
  Sum/1 -> Math Function/1
  Product/1 -> Sum/1
  Product1/1 -> Sum/2
  Product2/1 -> Sum/3
  Product3/1 -> Sum/4
  Demux/1 -> Product/2, Product/1
  Demux/2 -> Product1/2, Product1/1
  Demux/3 -> Product2/2, Product2/1
  Demux/4 -> Product3/2, Product3/1

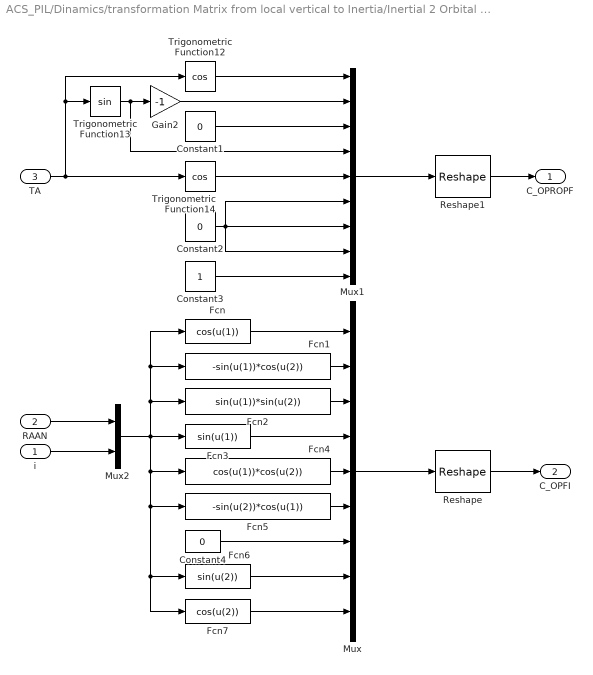
== system ACS_PIL/Dinamics/transformation Matrix from local vertical to Inertia/Inertial 2 Orbital Plane1 ==
  i : Inport
  RAAN : Inport  Port=2
  TA : Inport  Port=3
  Constant1 : Constant  Value=0
  Constant2 : Constant  Value=0
  Constant3 : Constant
  Constant4 : Constant  Value=0
  Fcn : Fcn  Expr=cos(u(1))
  Fcn1 : Fcn  Expr=-sin(u(1))*cos(u(2))
  Fcn2 : Fcn  Expr=sin(u(1))*sin(u(2))
  Fcn3 : Fcn  Expr=sin(u(1))
  Fcn4 : Fcn  Expr=cos(u(1))*cos(u(2))
  Fcn5 : Fcn  Expr=-sin(u(2))*cos(u(1))
  Fcn6 : Fcn  Expr=sin(u(2))
  Fcn7 : Fcn  Expr=cos(u(2))
  Gain2 : Gain  Gain=-1
  Mux : Mux  Inputs=9
  Mux1 : Mux  Inputs=9
  Mux2 : Mux  Inputs=2
  Reshape : Reshape  OutputDimensionality=Customize  OutputDimensions=[3,3]
  Reshape1 : Reshape  OutputDimensionality=Customize  OutputDimensions=[3,3]
  Trigonometric Function12 : Trigonometry  Operator=cos
  Trigonometric Function13 : Trigonometry
  Trigonometric Function14 : Trigonometry  Operator=cos
  C_OPROPF : Outport
  C_OPFI : Outport  Port=2
  wires:
  Reshape1/1 -> C_OPROPF/1
  Reshape/1 -> C_OPFI/1
  Fcn7/1 -> Mux/9
  Fcn6/1 -> Mux/8
  Constant4/1 -> Mux/7
  Fcn5/1 -> Mux/6
  Fcn4/1 -> Mux/5
  Fcn3/1 -> Mux/4
  Fcn2/1 -> Mux/3
  Fcn1/1 -> Mux/2
  Mux2/1 -> Fcn7/1, Fcn6/1, Fcn5/1, Fcn4/1, Fcn3/1, Fcn2/1, Fcn1/1, Fcn/1
  i/1 -> Mux2/2
  RAAN/1 -> Mux2/1
  Fcn/1 -> Mux/1
  TA/1 -> Trigonometric Function14/1, Trigonometric Function13/1, Trigonometric Function12/1
  Constant3/1 -> Mux1/9
  Constant2/1 -> Mux1/8, Mux1/7, Mux1/6
  Trigonometric Function14/1 -> Mux1/5
  Constant1/1 -> Mux1/3
  Gain2/1 -> Mux1/2
  Trigonometric Function13/1 -> Mux1/4, Gain2/1
  Trigonometric Function12/1 -> Mux1/1
  Mux1/1 -> Reshape1/1
  Mux/1 -> Reshape/1

== system ACS_PIL/Dinamics/transformation Matrix from local vertical to Inertia/Orbital Reference 2 Local Vertical1 ==
  Constant{,2..3,5..6,8} (6 alike) : Constant  Value=0
  Constant1 : Constant  Value=-1
  Constant4 : Constant  Value=-1
  Constant7 : Constant
  Mux : Mux  Inputs=9
  Reshape : Reshape  OutputDimensionality=Customize  OutputDimensions=[3,3]
  C_VOPR : Outport
  wires:
  Reshape/1 -> C_VOPR/1
  Constant6/1 -> Mux/9
  Constant4/1 -> Mux/8
  Constant8/1 -> Mux/7
  Constant5/1 -> Mux/6
  Constant/1 -> Mux/5
  Constant7/1 -> Mux/4
  Constant1/1 -> Mux/3
  Constant3/1 -> Mux/2
  Constant2/1 -> Mux/1
  Mux/1 -> Reshape/1

== system ACS_PIL/Earth/Simple model of Earth's Magnetic Field1/Simple model of Earth's Magnetic Field1 ==
  long : Inport
  lat : Inport  Port=2
  teta_md : Inport  Port=3
  phi_md : Inport  Port=4
  " 3nd gaussian coefficient1" : Constant  Value=2
  " 3nd gaussian coefficient4" : Constant
  Demux2 : Demux  Outputs=2
  Ground : Ground
  Ground1 : Ground
  Ground2 : Ground
  Inertial 2 Orbital Plane1 : Subsystem
  Mux : Mux  Inputs=2
  Mux4 : Mux  Inputs=2
  Mux5 : Mux  Inputs=2
  Simple Magnetc Field : Subsystem
  Sum : Sum
  Terminator{1..5} (5 alike) : Terminator
  dipole direction in geocentric inertial frame : Subsystem
  B_ECEF_T : Outport
  wires:
  dipole direction in geocentric inertial frame/1(Dipol_direction_ECEF) -> Simple Magnetc Field/1(dd_ECEF)
  phi_md/1 -> dipole direction in geocentric inertial frame/2(phi_md)
  teta_md/1 -> dipole direction in geocentric inertial frame/1(theta_md)
  long/1 -> Mux/1
  lat/1 -> Mux/2
  Simple Magnetc Field/1(B_NED) -> Mux5/1
  Simple Magnetc Field/2(B_ECEF) -> Mux5/2
  Demux2/1 -> Terminator5/1
  Demux2/2 -> B_ECEF_T/1
  Mux/1 -> Terminator2/1, Inertial 2 Orbital Plane1/1(long_lat)
  Inertial 2 Orbital Plane1/1(C_NED_ECEF) -> Simple Magnetc Field/2(C_NED_ECEF), Terminator1/1
  " 3nd gaussian coefficient4"/1 -> Simple Magnetc Field/Enable
  " 3nd gaussian coefficient1"/1 -> Terminator3/1
  Mux5/1 -> Sum/1
  Sum/1 -> Demux2/1
  Ground/1 -> Mux4/1
  Ground1/1 -> Mux4/2
  Mux4/1 -> Terminator4/1
  Ground2/1 -> Sum/2

== system ACS_PIL/Earth/Simple model of Earth's Magnetic Field1/longitude_latitude ==
  R_ECEF : Inport
  Constant2 : Constant  Value=r
  Demux : Demux  Outputs=3
  Mux : Mux  Inputs=2
  Product : Product  Inputs=*/  RndMeth=Zero
  Selector : Selector  InputPortWidth=3  IndexOptions=Index vector (dialog)  Indices=[2 1 3]  OutputSizes=1
  Trigonometric Function : Trigonometry  Operator=atan2
  Trigonometric Function1 : Trigonometry  Operator=asin
  long_lat : Outport
  wires:
  R_ECEF/1 -> Selector/1
  Trigonometric Function/1 -> Mux/1  "longitude"
  Demux/3 -> Product/1
  Constant2/1 -> Product/2
  Product/1 -> Trigonometric Function1/1
  Trigonometric Function1/1 -> Mux/2  "latitude"
  Mux/1 -> long_lat/1
  Selector/1 -> Demux/1
  Demux/1 -> Trigonometric Function/1
  Demux/2 -> Trigonometric Function/2

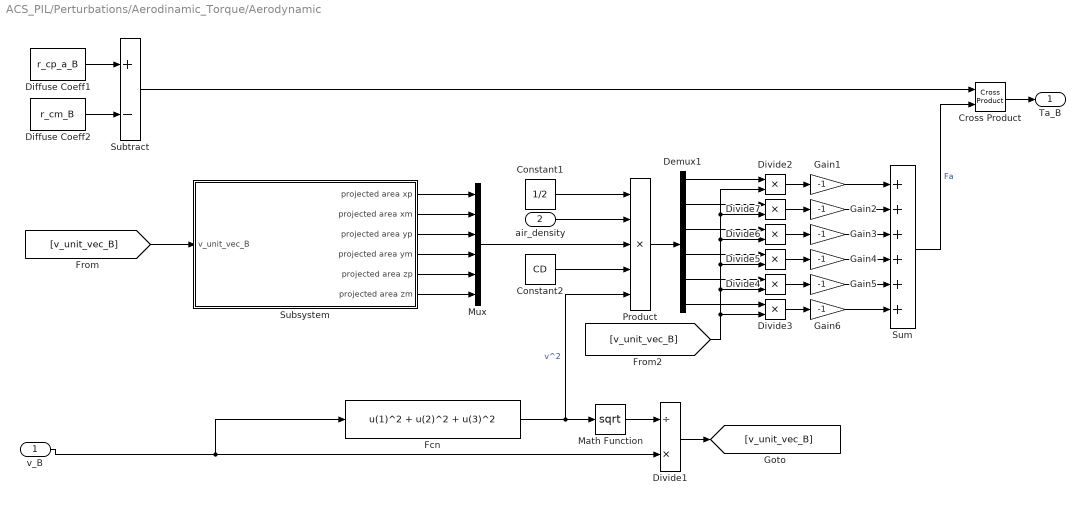
== system ACS_PIL/Perturbations/Aerodinamic_Torque/Aerodynamic ==
  v_B : Inport
  air_density : Inport  Port=2
  Constant1 : Constant  Value=1/2
  Constant2 : Constant  Value=CD
  Cross Product : vrlib/Utilities/Cross Product
      settings: SourceProductBaseCode=VR
  Demux1 : Demux  Outputs=6
  Diffuse Coeff1 : Constant  Value=r_cp_a_B
  Diffuse Coeff2 : Constant  Value=r_cm_B
  Divide1 : Product  Inputs=/*
  Divide{2..7} (6 alike) : Product  Inputs=**
  Fcn : Fcn  Expr=u(1)^2 + u(2)^2 + u(3)^2
  Gain{1..6} (6 alike) : Gain  Gain=-1
  Math Function : Math  Operator=sqrt  SaturateOnIntegerOverflow=on
  Mux : Mux  Inputs=6
  Product : Product  Inputs=5  RndMeth=Zero
  Subsystem : Subsystem
  Subtract : Sum  Inputs=+-
  Sum : Sum  Inputs=++++++
  Ta_B : Outport
  wires:
  v_B/1 -> Fcn/1, Divide1/2
  Constant1/1 -> Product/1
  air_density/1 -> Product/2
  Constant2/1 -> Product/4
  Fcn/1 -> Math Function/1, Product/5  "v^2"
  Math Function/1 -> Divide1/1
  Divide1/1 -> [v_unit_vec_B]
  [v_unit_vec_B] -> Subsystem/1(v_unit_vec_B)
  Subsystem/1(projected area xp) -> Mux/1
  Subsystem/2(projected area xm) -> Mux/2
  Subsystem/3(projected area yp) -> Mux/3
  Subsystem/4(projected area ym) -> Mux/4
  Subsystem/5(projected area zp) -> Mux/5
  Subsystem/6(projected area zm) -> Mux/6
  Mux/1 -> Product/3
  Sum/1 -> Cross Product/2  "Fa"
  Product/1 -> Demux1/1
  Demux1/1 -> Divide2/1
  [v_unit_vec_B] -> Divide3/2, Divide4/2, Divide5/2, Divide6/2, Divide7/2, Divide2/2
  Demux1/6 -> Divide3/1
  Demux1/5 -> Divide4/1
  Demux1/4 -> Divide5/1
  Demux1/3 -> Divide6/1
  Demux1/2 -> Divide7/1
  Divide2/1 -> Gain1/1
  Divide7/1 -> Gain2/1
  Divide6/1 -> Gain3/1
  Divide5/1 -> Gain4/1
  Divide4/1 -> Gain5/1
  Divide3/1 -> Gain6/1
  Gain1/1 -> Sum/1
  Gain2/1 -> Sum/2
  Gain3/1 -> Sum/3
  Gain4/1 -> Sum/4
  Gain5/1 -> Sum/5
  Gain6/1 -> Sum/6
  Diffuse Coeff1/1 -> Subtract/1
  Diffuse Coeff2/1 -> Subtract/2
  Subtract/1 -> Cross Product/1
  Cross Product/1 -> Ta_B/1

== system ACS_PIL/Perturbations/Aerodinamic_Torque/Subsystem ==
  C_BV : Inport
  Mux : Mux  Inputs=3
  Orbit angular velocity : Constant  Value=omega_o
  Product1 : Product  RndMeth=Zero
  Product2 : Product  Multiplication=Matrix(*)  RndMeth=Zero
  r_sat1 : Constant  Value=r
  r_sat2 : Constant  Value=0
  r_sat3 : Constant  Value=0
  v_vec_b : Outport
  wires:
  Product2/1 -> v_vec_b/1
  C_BV/1 -> Product2/1
  r_sat3/1 -> Mux/3
  r_sat2/1 -> Mux/2
  Mux/1 -> Product2/2
  Product1/1 -> Mux/1
  Orbit angular velocity/1 -> Product1/2
  r_sat1/1 -> Product1/1

== system ACS_PIL/Perturbations/perturbation_Torque1/Power Generated ==
  Sol_b_W : Inport
  Add : Sum  Inputs=+++
  Add1 : Sum  Inputs=2
  Compare To Zero : simulink/Logic and Bit Operations/Compare To Zero  relop===  OutDataTypeStr=uint8  ZeroCross=off
  Demux : Demux  Outputs=3
  Math Function : Math  Operator=magnitude^2  SaturateOnIntegerOverflow=on
  Math Function1 : Math  Operator=magnitude^2  SaturateOnIntegerOverflow=on
  Math Function2 : Math  Operator=magnitude^2  SaturateOnIntegerOverflow=on
  Math Function3 : Math  Operator=sqrt  SaturateOnIntegerOverflow=on
  Product4 : Product  Inputs=*/  RndMeth=Zero
  Solar_Direction_b : Outport
  Solar_Flux_W : Outport  Port=2
  wires:
  Compare To Zero/1 -> Add1/2
  Add1/1 -> Product4/2
  Product4/1 -> Solar_Direction_b/1
  Sol_b_W/1 -> Demux/1, Product4/1
  Math Function2/1 -> Add/3
  Demux/3 -> Math Function2/1
  Math Function3/1 -> Compare To Zero/1, Solar_Flux_W/1, Add1/1
  Add/1 -> Math Function3/1
  Math Function1/1 -> Add/2
  Math Function/1 -> Add/1
  Demux/2 -> Math Function1/1
  Demux/1 -> Math Function/1

== system ACS_PIL/Perturbations/perturbation_Torque1/Solar Torque and Force Calculation ==
  S_ES_B : Inport
  Solar_const : Inport  Port=2
  eclipse : Inport  Port=3
  Force_toque1 : Subsystem
  Product2 : Product  Inputs=**  RndMeth=Zero
  Surface-Sun Angle : Subsystem
  Ts_B : Outport
  wires:
  eclipse/1 -> Product2/2
  S_ES_B/1 -> Surface-Sun Angle/1(S_ES_B), Force_toque1/3(S_ES_B)
  Product2/1 -> Ts_B/1
  Force_toque1/1(Ts_B) -> Product2/1
  Solar_const/1 -> Force_toque1/1(Solar_const)
  Surface-Sun Angle/1(theta) -> Force_toque1/2(theta)

== system ACS_PIL/Sun1/Solar Rays Direction/Eclipse_ ==
  Earth-Sun B : Inport
  C_BV : Inport  Port=2
  Compare to : simulink/Logic and Bit Operations/Compare To Constant  relop=>  const=cos(AE)  OutDataTypeStr=uint8  ZeroCross=off
  Dot Product1 : DotProduct  InputSameDT=on  OutDataTypeStr=Inherit: Inherit via internal rule
  Product1 : Product  Multiplication=Matrix(*)  RndMeth=Zero
  norm : Subsystem
  norm1 : Subsystem
  sat_earth vector in local vertical reference system : Constant  Value=[0 ;0 ;1]  VectorParams1D=off
  eclipse : Outport
  wires:
  Product1/1 -> norm1/1(1)
  norm/1(2) -> Dot Product1/1  "sat-sun"
  Earth-Sun B/1 -> norm/1(1)
  norm1/1(2) -> Dot Product1/2  "sat-earth"
  Compare to/1 -> eclipse/1
  Dot Product1/1 -> Compare to/1  "cos alpha"
  sat_earth vector in local vertical reference system/1 -> Product1/2
  C_BV/1 -> Product1/1

== system ACS_PIL/Sun1/Solar Rays Direction/Solar direction in inertial ==
  delta : Inport
  epsilon : Inport  Port=2
  gamma : Inport  Port=3
  Divide : Product  Inputs=**  Multiplication=Matrix(*)
  Inertial 2 Orbital Plane1 : Subsystem  mask(Inertial 2 Mean Sun){}
      mask help:
      | This Block performs the transformation matrix using angle between vernal equinox and Earth-MeanSun (gamma) for transformation from Inertial coordinate frame to Mean Sun coordinate frame.
      | The origin of  Mean Sun coordinate frame is on Earth center and its x-axis is toward Mean Sun and its z-axis is toward Earth North Pole.
      | Where Mean Sun is a virtual Sun which is rotating around Earth in a circular orbit with 1 year period.
      |
      |             [  c(gamma)        S(gamma)     0 ]
      | C_MSI =[ -S(gamma)      C(gamma)      0 ]
      |              [  0                        0                 1 ]
      mask Display:
      | port_label('input', 1, '\gamma','texmode','on')
      | port_label('output', 1, 'C_I^{MS}','texmode','on')
      | disp('Inertial 2 Mean Sun')
  Math Function : Math  Operator=transpose  SaturateOnIntegerOverflow=on
  Mux : Mux  Inputs=3
  Product1 : Product  RndMeth=Zero
  Product2 : Product  RndMeth=Zero
  Trigonometric Function : Trigonometry  Operator=cos
  Trigonometric Function1 : Trigonometry  Operator=cos
  Trigonometric Function2 : Trigonometry  Operator=cos
  Trigonometric Function3 : Trigonometry
  Trigonometric Function4 : Trigonometry
  S_ES_I : Outport
  wires:
  Math Function/1 -> Divide/1
  gamma/1 -> Inertial 2 Orbital Plane1/1(gamma)
  Divide/1 -> S_ES_I/1
  Inertial 2 Orbital Plane1/1(C_MSI) -> Math Function/1
  Mux/1 -> Divide/2
  Trigonometric Function4/1 -> Mux/3
  Product1/1 -> Mux/2
  Product2/1 -> Mux/1
  Trigonometric Function1/1 -> Product2/2
  Trigonometric Function/1 -> Product2/1
  epsilon/1 -> Trigonometric Function1/1, Trigonometric Function3/1
  delta/1 -> Trigonometric Function4/1, Trigonometric Function/1, Trigonometric Function2/1
  Trigonometric Function2/1 -> Product1/1
  Trigonometric Function3/1 -> Product1/2
